simulink subsystem "wheel_inertia"  (R2024b)
settings: Solver=VariableStepAuto  StartTime=0.0  StopTime=10.0  RelTol=1e-3
model mask{radius=0, spin_inertia=0, initial_spin=0}
  mask prompts: radius "Wheel radius [m]"; spin_inertia "Wheel inertia [kg m^2]"; initial_spin "Initial spin [rad/s]"
settings Model: Creator=yevge  LastModifiedBy=yevge

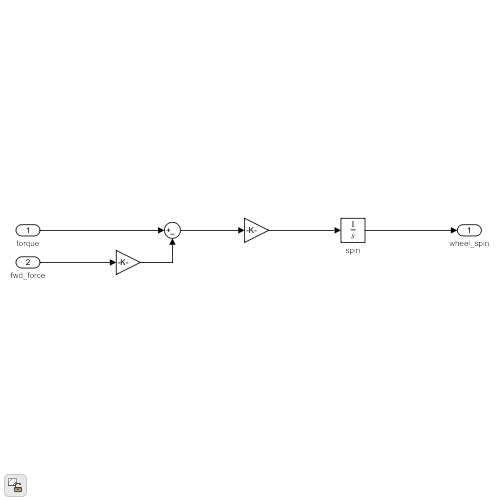
[thumbnail: Simulink's stored preview of the top-level diagram]
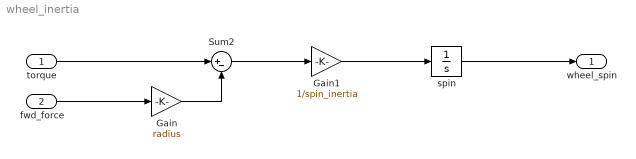
== system wheel_inertia ==
  torque : Inport
  fwd_force : Inport  Port=2
  Gain : Gain  Gain=radius
  Gain1 : Gain  Gain=1/spin_inertia
  Sum2 : Sum  Inputs=|+-
  spin : Integrator  InitialCondition=initial_spin  ContinuousStateAttributes='spin'
  wheel_spin : Outport
  wires:
  Sum2/1 -> Gain1/1
  torque/1 -> Sum2/1
  Gain/1 -> Sum2/2
  Gain1/1 -> spin/1
  fwd_force/1 -> Gain/1
  spin/1 -> wheel_spin/1
